simulink model "acHierarchicalStart"  (Simulink 7.2)
settings: Solver=VariableStepDiscrete  StartTime=0.0  StopTime=20  RelTol=1e-3
PreLoadFcn:
  | dT = 2;
settings Model: Creator=jrivitus  LastModifiedBy=jrivitus
settings OptimizationCC: EfficientMapNaN2IntZero=off

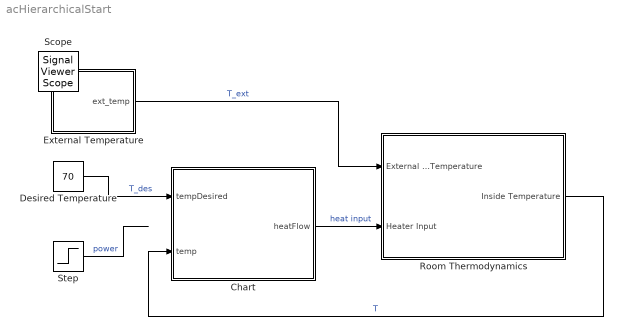
== system acHierarchicalStart ==
  Chart : Stateflow chart
  Desired Temperature : Constant  Value=70  OutDataType=sfix(16)  OutScaling=2^0
  External Temperature : Subsystem
  Room Thermodynamics : Subsystem
  Step : Step  Time=13  Before=1  After=0  SampleTime=0
  Scope : SignalViewerScope  IOType=viewer  NumInputPorts=2  RefreshTime=0.035000
      settings: TimeRange=20  YMin=50~-0.2  YMax=100~1.2
  wires:
  External Temperature/1(ext_temp) -> Room Thermodynamics/1(External Temperature)  "T_ext"
  Chart/1(heatFlow) -> Room Thermodynamics/2(Heater Input)  "heat input"
  Desired Temperature/1 -> Chart/1(tempDesired)  "T_des"
  Room Thermodynamics/1(Inside Temperature) -> Chart/2(temp)  "T"
  Step/1 -> ?  "power"

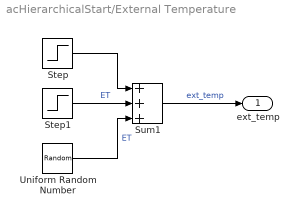
== system acHierarchicalStart/External Temperature ==
  Step : Step  Time=15  Before=70  After=40  SampleTime=0.1
  Step1 : Step  Time=5  After=20  SampleTime=0.1
  Sum1 : Sum  Inputs=+++  OutDataType=sfix(16)  OutScaling=2^0  SaturateOnIntegerOverflow=on
  Uniform Random Number : UniformRandomNumber  Minimum=-10  Maximum=10  SampleTime=0.1
  ext_temp : Outport
  wires:
  Step1/1 -> Sum1/2  "ET"
  Step/1 -> Sum1/1
  Uniform Random Number/1 -> Sum1/3  "ET"
  Sum1/1 -> ext_temp/1  "ext_temp"

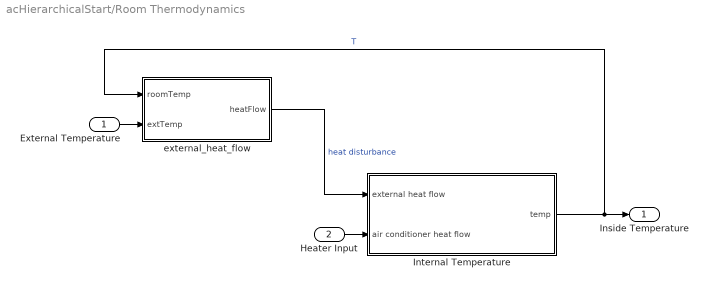
== system acHierarchicalStart/Room Thermodynamics ==
  External Temperature : Inport
  Heater Input : Inport  Port=2
  Internal Temperature : Subsystem
  external_heat_flow : Subsystem
  Inside Temperature : Outport
  wires:
  external_heat_flow/1(heatFlow) -> Internal Temperature/1(external heat flow)  "heat disturbance"
  Internal Temperature/1(temp) -> external_heat_flow/1(roomTemp), Inside Temperature/1  "T"
  External Temperature/1 -> external_heat_flow/2(extTemp)
  Heater Input/1 -> Internal Temperature/2(air conditioner heat flow)

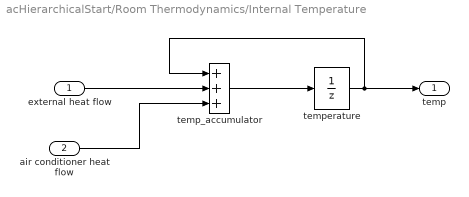
== system acHierarchicalStart/Room Thermodynamics/Internal Temperature ==
  external heat flow : Inport
  air conditioner heat flow : Inport  Port=2
  temp_accumulator : Sum  Inputs=+++  OutDataType=sfix(16)  OutScaling=2^-10
  temperature : UnitDelay  X0=70  SampleTime=0.1
  temp : Outport
  wires:
  air conditioner heat flow/1 -> temp_accumulator/3
  external heat flow/1 -> temp_accumulator/2
  temp_accumulator/1 -> temperature/1
  temperature/1 -> temp/1, temp_accumulator/1

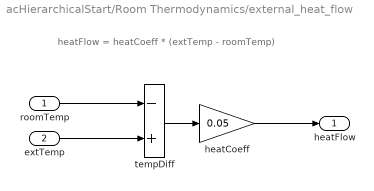
== system acHierarchicalStart/Room Thermodynamics/external_heat_flow ==
  note: heatFlow = heatCoeff * (extTemp - roomTemp)
  roomTemp : Inport  OutDataType=sfix(16)  OutScaling=2^0
  extTemp : Inport  Port=2  OutDataType=sfix(16)  OutScaling=2^0
  heatCoeff : Gain  Gain=0.05  ParameterDataType=sfix(16)  ParameterScaling=2^0  OutDataType=sfix(16)  OutScaling=2^0
  tempDiff : Sum  Inputs=-+  OutDataType=sfix(16)  OutScaling=2^-10
  heatFlow : Outport  DataType=double  OutDataType=sfix(16)  OutScaling=2^0  OutDataTypeStr=double  InitialOutput=0
  wires:
  extTemp/1 -> tempDiff/2
  roomTemp/1 -> tempDiff/1
  heatCoeff/1 -> heatFlow/1
  tempDiff/1 -> heatCoeff/1

== stateflow chart Chart ==
  state Off
    entry:
    heatFlow=0;
  state HeaterOn
    entry:
    heatFlow=1;
  state CoolerOn
    entry:
    heatFlow=-1;
  (default) -> Off
  Off -> HeaterOn [order 1] : [temp < (tempDesired-dT)]
  Off -> CoolerOn [order 2] : [temp > (tempDesired+dT)]
  HeaterOn -> Off : [temp > (tempDesired-dT)]
  CoolerOn -> Off : [temp < (tempDesired+dT)]
  data: tempDesired input double; heatFlow output double; temp input double; dT parameter double
